simulink model "fifth_07_03_25vs"  (R2024b)
settings: Solver=VariableStepAuto  StartTime=0.0  StopTime=10.0  MaxStep=1e-5  RelTol=1e-3
values from neighbouring files (symbols this model uses):
  fsw = 5e3    (= 5000)    [fifth_07_03_25_parameters.m]
  l = 1e-3    (= 0.001)    [fifth_07_03_25_parameters.m]
  r = 10    [fifth_07_03_25_parameters.m]
libraries: simulink x6
settings Model: Creator=Franco  LastModifiedBy=Franco

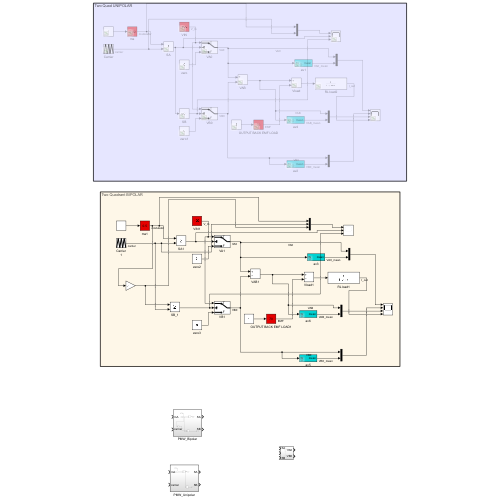
[thumbnail: Simulink's stored preview of the top-level diagram]
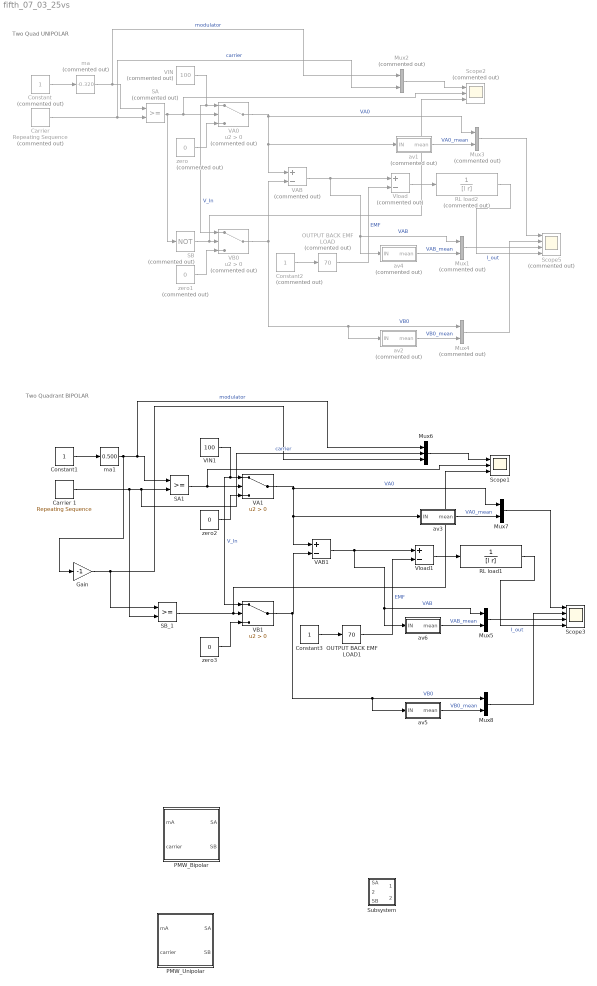
== system fifth_07_03_25vs ==
  note: Two Quadrant BIPOLAR
  note: Two Quad UNIPOLAR
  "Carrier " : simulink/Sources/Repeating Sequence  Commented=on  rep_seq_t=[0 0.5/fsw 1/fsw]  rep_seq_y=[-1 1 -1 ]
  Carrier 1 : simulink/Sources/Repeating Sequence  rep_seq_t=[0 0.5/fsw 1/fsw]  rep_seq_y=[-1 1 -1 ]
  Constant : Constant  Commented=on
  Constant1 : Constant
  Constant2 : Constant  Commented=on
  Constant3 : Constant
  Gain : Gain  Gain=-1
  Mux{1..4} (4 alike) : Mux  Commented=on  Inputs=2
  Mux5 : Mux  Inputs=2
  Mux6 : Mux  Inputs=3
  Mux7 : Mux  Inputs=2
  Mux8 : Mux  Inputs=2
  OUTPUT BACK EMF LOAD : simulink/Math Operations/Slider Gain  Commented=on  gain=70  low=0  high=100
  OUTPUT BACK EMF LOAD1 : simulink/Math Operations/Slider Gain  gain=70  low=0  high=100
  PMW_Bipolar : Subsystem
  PMW_Unipolar : Subsystem
  RL load1 : TransferFcn  Denominator=[l r]
  RL load2 : TransferFcn  Commented=on  Denominator=[l r]
  SA : RelationalOperator  Commented=on  OutDataTypeStr=boolean  RndMeth=Simplest  InputSameDT=off
  SA1 : RelationalOperator  OutDataTypeStr=boolean  RndMeth=Simplest  InputSameDT=off
  SB : Logic  Commented=on  Operator=NOT  AllPortsSameDT=off  OutDataTypeStr=boolean
  SB_1 : RelationalOperator  OutDataTypeStr=boolean  RndMeth=Simplest  InputSameDT=off
  Scope1 : Scope  NumInputPorts=3
  Scope2 : Scope  Commented=on  NumInputPorts=3
  Scope3 : Scope  NumInputPorts=4
  Scope5 : Scope  Commented=on  NumInputPorts=4
  Subsystem : Subsystem
  VA0 : Switch  Commented=on  Criteria=u2 > Threshold  SaturateOnIntegerOverflow=off  InputSameDT=off
  VA1 : Switch  Criteria=u2 > Threshold  SaturateOnIntegerOverflow=off  InputSameDT=off
  VAB : Sum  Commented=on  Inputs=+-
  VAB1 : Sum  Inputs=+-
  VB0 : Switch  Commented=on  Criteria=u2 > Threshold  SaturateOnIntegerOverflow=off  InputSameDT=off
  VB1 : Switch  Criteria=u2 > Threshold  SaturateOnIntegerOverflow=off  InputSameDT=off
  VIN : Constant  Commented=on  Value=100
  VIN1 : Constant  Value=100
  Vload : Sum  Commented=on  Inputs=+-
  Vload1 : Sum  Inputs=+-
  av1 : Subsystem  Commented=on  mask{period=1/fsw}
      mask prompts: period "period [s]"
      mask DialogControl DescTextVar Prompt: calculate the averge over period
      mask DialogControl text Prompt: test
  av2 : Subsystem  Commented=on  mask{period=1/fsw}
      mask prompts: period "period [s]"
      mask DialogControl DescTextVar Prompt: calculate the averge over period
      mask DialogControl text Prompt: test
  av3 : Subsystem  mask{period=1/fsw}
      mask prompts: period "period [s]"
      mask DialogControl DescTextVar Prompt: calculate the averge over period
      mask DialogControl text Prompt: test
  av4 : Subsystem  Commented=on  mask{period=1/fsw}
      mask prompts: period "period [s]"
      mask DialogControl DescTextVar Prompt: calculate the averge over period
      mask DialogControl text Prompt: test
  av5 : Subsystem  mask{period=1/fsw}
      mask prompts: period "period [s]"
      mask DialogControl DescTextVar Prompt: calculate the averge over period
      mask DialogControl text Prompt: test
  av6 : Subsystem  mask{period=1/fsw}
      mask prompts: period "period [s]"
      mask DialogControl DescTextVar Prompt: calculate the averge over period
      mask DialogControl text Prompt: test
  ma : simulink/Math Operations/Slider Gain  Commented=on  gain=-0.320  low=-1  high=1
  ma1 : simulink/Math Operations/Slider Gain  gain=0.500  low=-1  high=1
  zero : Constant  Commented=on  Value=0
  zero1 : Constant  Commented=on  Value=0
  zero2 : Constant  Value=0
  zero3 : Constant  Value=0
  wires:
  ma/1 -> Mux2/1, SA/1  "modulator"
  Constant/1 -> ma/1
  "Carrier "/1 -> Mux2/2, SA/2  "carrier"
  VIN/1 -> VB0/1, VA0/1  "V_In"
  SA/1 -> Scope2/2, VA0/2, SB/1
  zero/1 -> VA0/3
  zero1/1 -> VB0/3
  SB/1 -> Scope2/3, VB0/2
  VA0/1 -> Mux3/1, av1/1(IN), VAB/1  "VA0"
  VB0/1 -> av2/1(IN), Mux4/1, VAB/2  "VB0"
  VAB/1 -> Mux1/1, av4/1(IN), Vload/1  "VAB"
  Constant2/1 -> OUTPUT BACK EMF LOAD/1
  Vload/1 -> RL load2/1
  OUTPUT BACK EMF LOAD/1 -> Vload/2  "EMF"
  Mux2/1 -> Scope2/1
  av4/1(mean) -> Mux1/2  "VAB_mean"
  Mux1/1 -> Scope5/3
  Mux3/1 -> Scope5/1
  av1/1(mean) -> Mux3/2  "VA0_mean"
  Mux4/1 -> Scope5/2
  av2/1(mean) -> Mux4/2  "VB0_mean"
  RL load2/1 -> Scope5/4  "I_out"
  RL load1/1 -> Scope3/4  "I_out"
  av5/1(mean) -> Mux8/2  "VB0_mean"
  Mux8/1 -> Scope3/2
  av3/1(mean) -> Mux7/2  "VA0_mean"
  Mux7/1 -> Scope3/1
  Mux5/1 -> Scope3/3
  av6/1(mean) -> Mux5/2  "VAB_mean"
  Mux6/1 -> Scope1/1
  OUTPUT BACK EMF LOAD1/1 -> Vload1/2  "EMF"
  Vload1/1 -> RL load1/1
  Constant3/1 -> OUTPUT BACK EMF LOAD1/1
  VAB1/1 -> Vload1/1, av6/1(IN), Mux5/1  "VAB"
  VB1/1 -> VAB1/2, Mux8/1, av5/1(IN)  "VB0"
  VA1/1 -> VAB1/1, av3/1(IN), Mux7/1  "VA0"
  SB_1/1 -> VB1/2, Scope1/3
  zero3/1 -> VB1/3
  zero2/1 -> VA1/3
  SA1/1 -> VA1/2, Scope1/2
  VIN1/1 -> VA1/1, VB1/1  "V_In"
  Carrier 1/1 -> SB_1/2, SA1/2, Mux6/2  "carrier"
  Constant1/1 -> ma1/1
  ma1/1 -> Gain/1, SA1/1, Mux6/1  "modulator"
  Gain/1 -> SB_1/1, Mux6/3

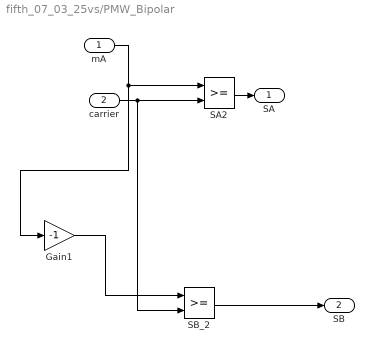
== system fifth_07_03_25vs/PMW_Bipolar ==
  mA : Inport
  carrier : Inport  Port=2
  Gain1 : Gain  Gain=-1
  SA2 : RelationalOperator  OutDataTypeStr=boolean  RndMeth=Simplest  InputSameDT=off
  SB_2 : RelationalOperator  OutDataTypeStr=boolean  RndMeth=Simplest  InputSameDT=off
  SA : Outport
  SB : Outport  Port=2
  wires:
  Gain1/1 -> SB_2/1
  mA/1 -> SA2/1, Gain1/1
  SA2/1 -> SA/1
  carrier/1 -> SB_2/2, SA2/2
  SB_2/1 -> SB/1

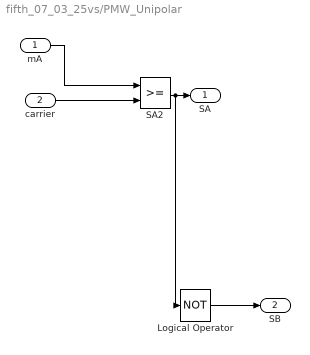
== system fifth_07_03_25vs/PMW_Unipolar ==
  mA : Inport
  carrier : Inport  Port=2
  Logical Operator : Logic  Operator=NOT  AllPortsSameDT=off  OutDataTypeStr=boolean
  SA2 : RelationalOperator  OutDataTypeStr=boolean  RndMeth=Simplest  InputSameDT=off
  SA : Outport
  SB : Outport  Port=2
  wires:
  carrier/1 -> SA2/2
  SA2/1 -> Logical Operator/1, SA/1
  mA/1 -> SA2/1
  Logical Operator/1 -> SB/1

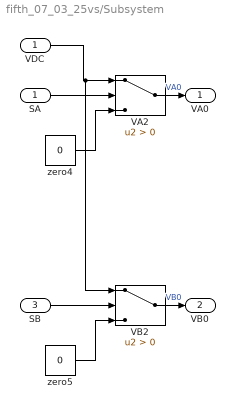
== system fifth_07_03_25vs/Subsystem ==
  SA : Inport
  SB : Inport  Port=3
  VA2 : Switch  Criteria=u2 > Threshold  SaturateOnIntegerOverflow=off  InputSameDT=off
  VB2 : Switch  Criteria=u2 > Threshold  SaturateOnIntegerOverflow=off  InputSameDT=off
  VDC : InportShadow
  zero4 : Constant  Value=0
  zero5 : Constant  Value=0
  VA0 : Outport
  VB0 : Outport  Port=2
  wires:
  SA/1 -> VA2/2
  zero4/1 -> VA2/3
  VB2/1 -> VB0/1  "VB0"
  SB/1 -> VB2/2
  zero5/1 -> VB2/3
  VA2/1 -> VA0/1  "VA0"
  VDC/1 -> VB2/1, VA2/1

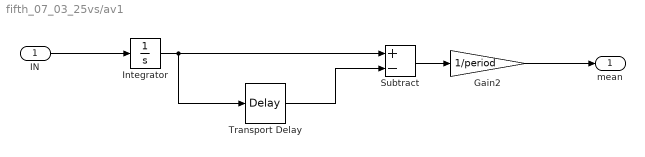
== system fifth_07_03_25vs/av1 ==
  IN : Inport
  Gain2 : Gain  Gain=1/period
  Integrator : Integrator
  Subtract : Sum  Inputs=+-
  Transport Delay : TransportDelay  DelayTime=period
  mean : Outport
  wires:
  IN/1 -> Integrator/1
  Transport Delay/1 -> Subtract/2
  Subtract/1 -> Gain2/1
  Gain2/1 -> mean/1
  Integrator/1 -> Subtract/1, Transport Delay/1

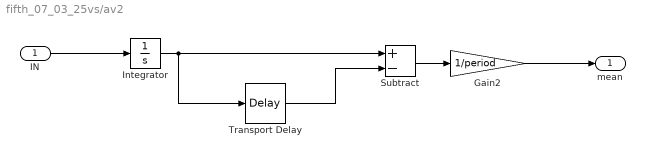
== system fifth_07_03_25vs/av2 ==
  IN : Inport
  Gain2 : Gain  Gain=1/period
  Integrator : Integrator
  Subtract : Sum  Inputs=+-
  Transport Delay : TransportDelay  DelayTime=period
  mean : Outport
  wires:
  IN/1 -> Integrator/1
  Transport Delay/1 -> Subtract/2
  Subtract/1 -> Gain2/1
  Gain2/1 -> mean/1
  Integrator/1 -> Subtract/1, Transport Delay/1

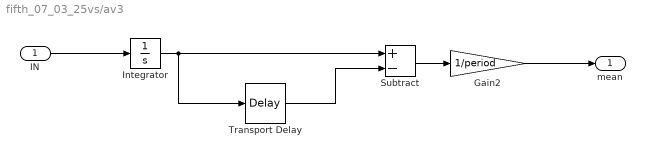
== system fifth_07_03_25vs/av3 ==
  IN : Inport
  Gain2 : Gain  Gain=1/period
  Integrator : Integrator
  Subtract : Sum  Inputs=+-
  Transport Delay : TransportDelay  DelayTime=period
  mean : Outport
  wires:
  Integrator/1 -> Transport Delay/1, Subtract/1
  Gain2/1 -> mean/1
  Subtract/1 -> Gain2/1
  Transport Delay/1 -> Subtract/2
  IN/1 -> Integrator/1

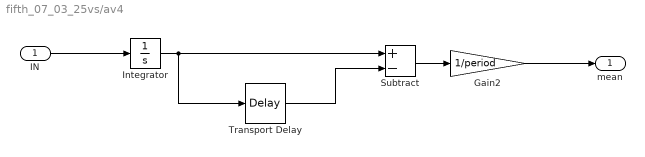
== system fifth_07_03_25vs/av4 ==
  IN : Inport
  Gain2 : Gain  Gain=1/period
  Integrator : Integrator
  Subtract : Sum  Inputs=+-
  Transport Delay : TransportDelay  DelayTime=period
  mean : Outport
  wires:
  Integrator/1 -> Transport Delay/1, Subtract/1
  Gain2/1 -> mean/1
  Subtract/1 -> Gain2/1
  Transport Delay/1 -> Subtract/2
  IN/1 -> Integrator/1

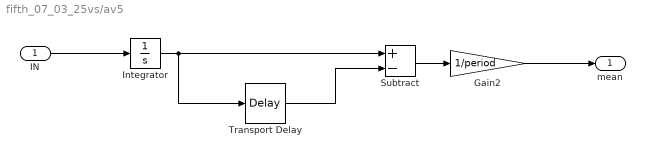
== system fifth_07_03_25vs/av5 ==
  IN : Inport
  Gain2 : Gain  Gain=1/period
  Integrator : Integrator
  Subtract : Sum  Inputs=+-
  Transport Delay : TransportDelay  DelayTime=period
  mean : Outport
  wires:
  Integrator/1 -> Transport Delay/1, Subtract/1
  Gain2/1 -> mean/1
  Subtract/1 -> Gain2/1
  Transport Delay/1 -> Subtract/2
  IN/1 -> Integrator/1

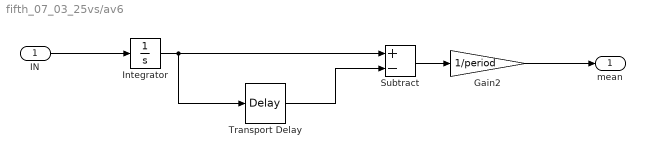
== system fifth_07_03_25vs/av6 ==
  IN : Inport
  Gain2 : Gain  Gain=1/period
  Integrator : Integrator
  Subtract : Sum  Inputs=+-
  Transport Delay : TransportDelay  DelayTime=period
  mean : Outport
  wires:
  IN/1 -> Integrator/1
  Transport Delay/1 -> Subtract/2
  Subtract/1 -> Gain2/1
  Gain2/1 -> mean/1
  Integrator/1 -> Subtract/1, Transport Delay/1
